simulink model "main_sim_adapt_Gref_SPPH"  (Simulink 7.2)
settings: Solver=ode2  SolverMode=SingleTasking  StartTime=0.0  StopTime=tsim_max  FixedStep=dtsim  RelTol=1e-3
StopFcn:
  | %mkplt
values from neighbouring files (symbols this model uses):
  assertion_time = inf    [setup_taem_sgs_al.m]
  cosA = cos(rwyAZ_rad)    [setup_taem_sgs_al.m]
  E_rwy = E_origin + (mod(( rwyLLA(2)/constants.r2d - lon_origin )+pi,2*pi)-pi) * constants.earth_radius * cos(lat_origin)    [setup_taem_sgs_al.m]
  eow_boundary = tmp_eow(ix(1))    [setup_taem_sgs_al.m]
  N_rwy = N_origin + (mod(( rwyLLA(1)/constants.r2d - lat_origin )+pi,2*pi)-pi) * constants.earth_radius    [setup_taem_sgs_al.m]
  sinA = sin(rwyAZ_rad)    [setup_taem_sgs_al.m]
  vel = 487.2512    [doit.m]
undefined symbols (not defined in the file or in its folder): accel_cmd, aero_surf_qbar_off, aero_surf_qbar_on, Alon, att_cmd_select, att_trim_IC, att_type, att_type_numbers, B1, bb_ellipsoid, bb_params, Blon, C, CA, chi_trim_IC, Clon, command_time, compute_all_rate_cols, compute_all_vel_cols, constants, da_trim_IC, dc_L2W_IC, de_trim_IC, DiscIntNeverNeededParam, dr_trim_IC, dtsim, DZkx, DZtheta, E_trim_IC, Ed_cmd, Ed_trim_IC, fc, flag_uad, full_surf_llim, full_surf_ulim, gain_set, gain_var_struct, gam_cmd_descent, gam_cmd_preflare, gamdot_cmd_descent, gamdot_cmd_flare, gamdot_cmd_preflare, gamma_trim_IC, Gamtheta, Gamx, h_trim_IC, hd_cmd, hd_trim_IC, ideal_vel_Kb, in_exsig_vecin, in_exsig_vecout, invCB, Kb, Kxhat0, Kxnom, Kxstar, lonxm0, MACH, MACH_att_fb, MACH_att_int_IC ... (+77)
libraries: simulink x36, utility_lib x36, mach_lib x24, model_lib x15, simulink_need_slupdate x8, models x6
(part 3 of 7)

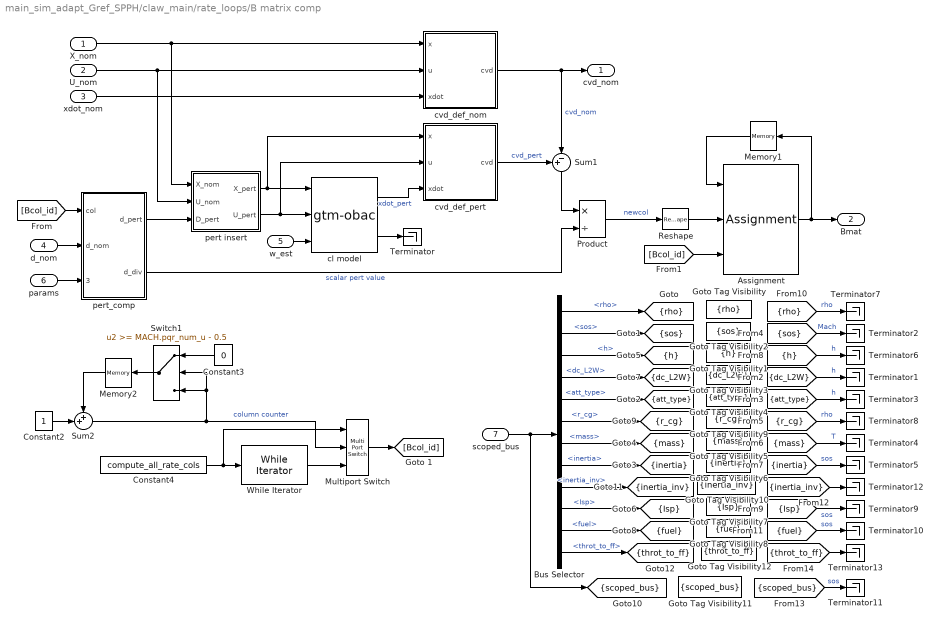
== system main_sim_adapt_Gref_SPPH/claw_main/rate_loops/B matrix comp ==
  X_nom : Inport  OutDataType=sfix(16)  OutScaling=2^0
  U_nom : Inport  Port=2  OutDataType=sfix(16)  OutScaling=2^0
  xdot_nom : Inport  Port=3  OutDataType=sfix(16)  OutScaling=2^0
  d_nom : Inport  Port=4  OutDataType=sfix(16)  OutScaling=2^0
  w_est : Inport  Port=5  OutDataType=sfix(16)  OutScaling=2^0
  params : Inport  Port=6  OutDataType=sfix(16)  OutScaling=2^0
  scoped_bus : Inport  Port=7  OutDataType=sfix(16)  OutScaling=2^0
  Assignment : Assignment  NumberOfDimensions=2  IndexOptions=Assign all,Index vector (port)  Indices=-1,1  OutputSizes=1,1
  Bus Selector : BusSelector  OutputSignals=atmos_env.rho,atmos_env.sos,atmos_env.h,dc_L2W,att_type,mass_props.r_cg,mass_props.mass,mass_props.inertia,mass_props.inertia_inv,mass_props.Isp,mass_props.fuel,mass_props.throt_to_ff
  Constant2 : Constant  OutDataType=sfix(16)  OutScaling=2^0
  Constant3 : Constant  Orientation=left  Value=0  OutDataType=sfix(16)  OutScaling=2^0
  Constant4 : Constant  Value=compute_all_rate_cols  OutDataType=sfix(16)  OutScaling=2^0
  Goto Tag Visibility : GotoTagVisibility  GotoTag=rho
  Goto Tag Visibility1 : GotoTagVisibility  GotoTag=h
  Goto Tag Visibility10 : GotoTagVisibility  GotoTag=inertia_inv
  Goto Tag Visibility11 : GotoTagVisibility  GotoTag=scoped_bus
  Goto Tag Visibility12 : GotoTagVisibility  GotoTag=throt_to_ff
  Goto Tag Visibility2 : GotoTagVisibility  GotoTag=sos
  Goto Tag Visibility3 : GotoTagVisibility  GotoTag=dc_L2W
  Goto Tag Visibility4 : GotoTagVisibility  GotoTag=att_type
  Goto Tag Visibility5 : GotoTagVisibility  GotoTag=mass
  Goto Tag Visibility6 : GotoTagVisibility  GotoTag=inertia
  Goto Tag Visibility7 : GotoTagVisibility  GotoTag=Isp
  Goto Tag Visibility8 : GotoTagVisibility  GotoTag=fuel
  Goto Tag Visibility9 : GotoTagVisibility  GotoTag=r_cg
  Memory1 : Memory  Orientation=left  X0=MACH_pqr_Bmat_IC  InheritSampleTime=on
  Memory2 : Memory  Orientation=left  InheritSampleTime=on
  Multiport Switch : MultiPortSwitch  Inputs=2  zeroidx=on
  Product : Product  Inputs=*/  OutDataType=sfix(16)  OutScaling=2^0  SaturateOnIntegerOverflow=on  InputSameDT=on  OutDataTypeStr=Inherit: Same as first input
  Reshape : Reshape  OutputDimensionality=Column vector (2-D)
  Sum1 : Sum  Orientation=down  Inputs=+-|  OutDataType=sfix(16)  OutScaling=2^0  SaturateOnIntegerOverflow=on  InputSameDT=on  OutDataTypeStr=Inherit: Same as first input
  Sum2 : Sum  Inputs=++|  OutDataType=sfix(16)  OutScaling=2^0  SaturateOnIntegerOverflow=on  InputSameDT=on  OutDataTypeStr=Inherit: Same as first input
  Switch1 : Switch  Orientation=left  Threshold=MACH.pqr_num_u - 0.5  SaturateOnIntegerOverflow=on  InputSameDT=on
  Terminator{,1..13} (14 alike) : Terminator
  While Iterator : WhileIterator  MaxIters=MACH.pqr_num_u  WhileBlockType=do-while  ShowIterationPort=on
  cl model : models/gtm-obac  SystemSampleTime=-1
  cvd_def_nom : Subsystem
  cvd_def_pert : Subsystem
  pert insert : Subsystem
  pert_comp : Subsystem
  cvd_nom : Outport  OutDataType=sfix(16)  OutScaling=2^0
  Bmat : Outport  Port=2  OutDataType=sfix(16)  OutScaling=2^0
  tag scope: Isp=scoped, att_type=scoped, dc_L2W=scoped, fuel=scoped, h=scoped, inertia=scoped, inertia_inv=scoped, mass=scoped, r_cg=scoped, rho=scoped, scoped_bus=scoped, sos=scoped, throt_to_ff=scoped
  wires:
  Reshape/1 -> Assignment/2
  pert_comp/1(d_pert) -> pert insert/3(D_pert)
  pert insert/1(X_pert) -> cvd_def_pert/1(x), cl model/1
  pert insert/2(U_pert) -> cvd_def_pert/2(u), cl model/2
  pert_comp/2(d_div) -> Product/2  "scalar pert value"
  [Bcol_id] -> pert_comp/1(col)
  Assignment/1 -> Bmat/1, Memory1/1
  [Bcol_id] -> Assignment/3
  Sum1/1 -> Product/1
  Product/1 -> Reshape/1  "newcol"
  X_nom/1 -> cvd_def_nom/1(x), pert insert/1(X_nom)
  U_nom/1 -> cvd_def_nom/2(u), pert insert/2(U_nom)
  xdot_nom/1 -> cvd_def_nom/3(xdot)
  cvd_def_pert/1(cvd) -> Sum1/1  "cvd_pert"
  cvd_def_nom/1(cvd) -> Sum1/2, cvd_nom/1  "cvd_nom"
  cl model/1 -> cvd_def_pert/3(xdot)  "xdot_pert"
  w_est/1 -> cl model/3
  d_nom/1 -> pert_comp/2(d_nom)
  Memory1/1 -> Assignment/1
  cl model/2 -> Terminator/1
  params/1 -> pert_comp/3(params)
  Constant4/1 -> Multiport Switch/1, While Iterator/1
  While Iterator/1 -> Multiport Switch/3
  Constant3/1 -> Switch1/1
  Sum2/1 -> Switch1/3, Switch1/2, Multiport Switch/2  "column counter"
  Switch1/1 -> Memory2/1
  Memory2/1 -> Sum2/1
  Constant2/1 -> Sum2/2
  Multiport Switch/1 -> [Bcol_id]
  scoped_bus/1 -> Bus Selector/1, [scoped_bus]
  [rho] -> Terminator7/1  "rho"
  [sos] -> Terminator2/1  "Mach"
  [h] -> Terminator6/1  "h"
  Bus Selector/1 -> [rho]  "<rho>"
  Bus Selector/2 -> [sos]  "<sos>"
  Bus Selector/3 -> [h]  "<h>"
  [dc_L2W] -> Terminator1/1  "h"
  Bus Selector/4 -> [dc_L2W]  "<dc_L2W>"
  [att_type] -> Terminator3/1  "h"
  Bus Selector/5 -> [att_type]  "<att_type>"
  [r_cg] -> Terminator8/1  "rho"
  [mass] -> Terminator4/1  "T"
  [inertia] -> Terminator5/1  "sos"
  Bus Selector/6 -> [r_cg]  "<r_cg>"
  Bus Selector/7 -> [mass]  "<mass>"
  Bus Selector/8 -> [inertia]  "<inertia>"
  [Isp] -> Terminator9/1  "sos"
  Bus Selector/10 -> [Isp]  "<Isp>"
  [fuel] -> Terminator10/1  "sos"
  Bus Selector/11 -> [fuel]  "<fuel>"
  [inertia_inv] -> Terminator12/1
  Bus Selector/9 -> [inertia_inv]  "<inertia_inv>"
  [scoped_bus] -> Terminator11/1  "sos"
  [throt_to_ff] -> Terminator13/1
  Bus Selector/12 -> [throt_to_ff]  "<throt_to_ff>"

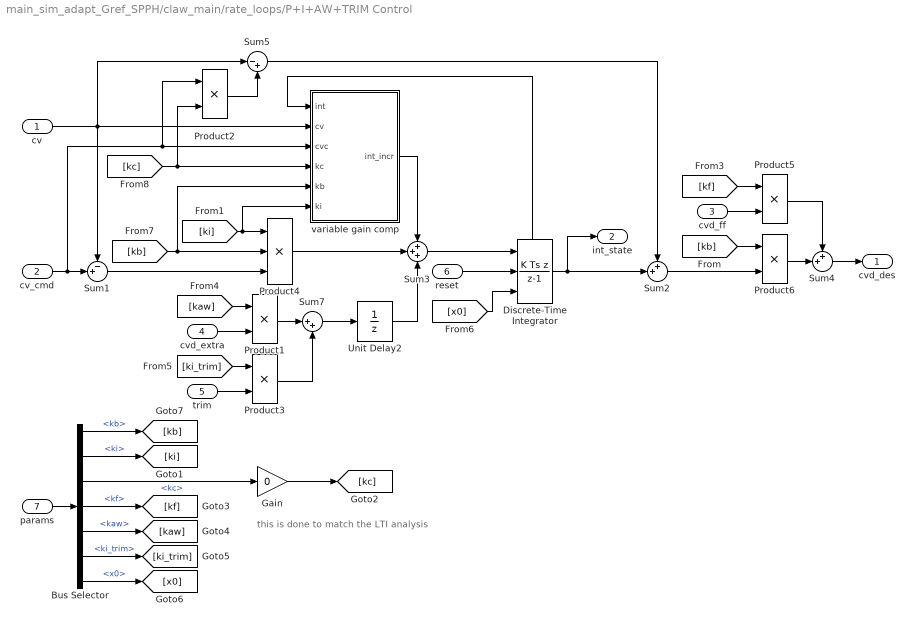
== system main_sim_adapt_Gref_SPPH/claw_main/rate_loops/P+I+AW+TRIM Control ==
  note: this is done to match the LTI analysis
  cv : Inport  OutDataType=sfix(16)  OutScaling=2^0
  cv_cmd : Inport  Port=2  OutDataType=sfix(16)  OutScaling=2^0
  cvd_ff : Inport  Port=3  OutDataType=sfix(16)  OutScaling=2^0
  cvd_extra : Inport  Port=4  OutDataType=sfix(16)  OutScaling=2^0
  trim : Inport  Port=5  OutDataType=sfix(16)  OutScaling=2^0
  reset : Inport  Port=6  OutDataType=sfix(16)  OutScaling=2^0
  params : Inport  Port=7  OutDataType=sfix(16)  OutScaling=2^0
  Bus Selector : BusSelector  OutputSignals=kb,ki,kc,kf,kaw,ki_trim,x0
  Discrete-Time Integrator : DiscreteIntegrator  IntegratorMethod=Integration: Backward Euler  ExternalReset=rising  InitialConditionSource=external  SampleTime=-1  OutDataType=sfix(16)  OutScaling=2^0  ShowStatePort=on  ICPrevOutput=DiscIntNeverNeededParam  ICPrevScaledInput=DiscIntNeverNeededParam
  Gain : Gain  Gain=0  ParameterDataType=sfix(16)  ParameterScaling=2^0  OutDataType=sfix(16)  OutScaling=2^0
  Product{1..3,5..6} (5 alike) : Product  OutDataType=sfix(16)  OutScaling=2^0  RndMeth=Zero
  Product4 : Product  Inputs=3  OutDataType=sfix(16)  OutScaling=2^0  RndMeth=Zero
  Sum1 : Sum  Inputs=-+|  OutDataType=sfix(16)  OutScaling=2^0  SaturateOnIntegerOverflow=on  InputSameDT=on  OutDataTypeStr=Inherit: Same as first input
  Sum2 : Sum  Inputs=++|  OutDataType=sfix(16)  OutScaling=2^0  SaturateOnIntegerOverflow=on  InputSameDT=on  OutDataTypeStr=Inherit: Same as first input
  Sum3 : Sum  Inputs=+++  OutDataType=sfix(16)  OutScaling=2^0  SaturateOnIntegerOverflow=on  InputSameDT=on  OutDataTypeStr=Inherit: Same as first input
  Sum4 : Sum  Inputs=++|  OutDataType=sfix(16)  OutScaling=2^0  SaturateOnIntegerOverflow=on  InputSameDT=on  OutDataTypeStr=Inherit: Same as first input
  Sum5 : Sum  Inputs=|-+  OutDataType=sfix(16)  OutScaling=2^0  SaturateOnIntegerOverflow=on  InputSameDT=on  OutDataTypeStr=Inherit: Same as first input
  Sum7 : Sum  Inputs=|++  OutDataType=sfix(16)  OutScaling=2^0  SaturateOnIntegerOverflow=on  InputSameDT=on  OutDataTypeStr=Inherit: Same as first input
  Unit Delay2 : UnitDelay  SampleTime=-1
  variable gain comp : Subsystem
  cvd_des : Outport  OutDataType=sfix(16)  OutScaling=2^0
  int_state : Outport  Port=2  OutDataType=sfix(16)  OutScaling=2^0
  wires:
  cv_cmd/1 -> Sum1/2, Product2/1, variable gain comp/3(cvc)
  [kb] -> variable gain comp/5(kb), Product4/2
  Sum5/1 -> Sum2/1
  Product2/1 -> Sum5/2
  [kc] -> Product2/2, variable gain comp/4(kc)
  Discrete-Time Integrator/State -> variable gain comp/1(int)
  variable gain comp/1(int_incr) -> Sum3/1
  Product4/1 -> Sum3/2
  Sum2/1 -> Product6/2
  cv/1 -> variable gain comp/2(cv), Sum5/1, Sum1/1
  Bus Selector/7 -> [x0]  "<x0>"
  params/1 -> Bus Selector/1
  [kf] -> Product5/1
  cvd_ff/1 -> Product5/2
  [kb] -> Product6/1
  [ki] -> variable gain comp/6(ki), Product4/1
  Sum1/1 -> Product4/3
  [ki_trim] -> Product3/1
  Product1/1 -> Sum7/1
  [kaw] -> Product1/1
  Bus Selector/6 -> [ki_trim]  "<ki_trim>"
  Bus Selector/5 -> [kaw]  "<kaw>"
  Bus Selector/4 -> [kf]  "<kf>"
  Bus Selector/3 -> Gain/1  "<kc>"
  Bus Selector/2 -> [ki]  "<ki>"
  Bus Selector/1 -> [kb]  "<kb>"
  Sum7/1 -> Unit Delay2/1
  Product3/1 -> Sum7/2
  reset/1 -> Discrete-Time Integrator/2
  cvd_extra/1 -> Product1/2
  Discrete-Time Integrator/1 -> Sum2/2, int_state/1
  Sum3/1 -> Discrete-Time Integrator/1
  Unit Delay2/1 -> Sum3/3
  trim/1 -> Product3/2
  Product6/1 -> Sum4/2
  Sum4/1 -> cvd_des/1
  Product5/1 -> Sum4/1
  [x0] -> Discrete-Time Integrator/3
  Gain/1 -> [kc]

== system main_sim_adapt_Gref_SPPH/claw_main/rate_loops/allocation ==
  cvd_nom : Inport  OutDataType=sfix(16)  OutScaling=2^0
  Bmat : Inport  Port=2  OutDataType=sfix(16)  OutScaling=2^0
  d_old : Inport  Port=3  OutDataType=sfix(16)  OutScaling=2^0
  d_nom : Inport  Port=4  OutDataType=sfix(16)  OutScaling=2^0
  cvd_des : Inport  Port=5  OutDataType=sfix(16)  OutScaling=2^0
  params : Inport  Port=6  OutDataType=sfix(16)  OutScaling=2^0
  Bmat_rcs : Selector  NumberOfDimensions=2  InputPortWidth=MACH.num_u  IndexOptions=Select all,Index vector (dialog)  Indices=-1,MACH.pqr_u_rcs_idx  OutputSizes=1
  Bmat_smn : Selector  NumberOfDimensions=2  InputPortWidth=MACH.num_u  IndexOptions=Select all,Index vector (dialog)  Indices=-1,MACH.pqr_u_smn_idx  OutputSizes=1
  Gain : Gain  Gain=-1  ParameterDataType=sfix(16)  ParameterScaling=2^0  OutDataType=sfix(16)  OutScaling=2^0
  Mux3 : Mux  Inputs=2
  RCS allocation : Subsystem
  Selector : Selector  NumberOfDimensions=2  InputPortWidth=MACH.num_u  IndexOptions=Index vector (dialog),Index vector (dialog)  Indices=1:9,1:2  OutputSizes=1
  config_di : Subsystem  BlockChoice=di_smn  mask{num_cv=MACH.pqr_num_cv, num_u=MACH.pqr_num_u_smn, wght_cv_type=MACH.pqr_wght_cv_type}
      link override di_smn/config_smn/smn_sfunc: sfunc_name=MACH.smn_sfunc_name
      settings: AttributesFormatString=%<BlockChoice>  TemplateBlock=mach_lib/config_di  MemberBlocks=di_pseudoinv,di_smn
  d_nom_smn : Selector  InputPortWidth=MACH.pqr_num_u  IndexOptions=Index vector (dialog)  Indices=MACH.pqr_u_smn_idx  OutputSizes=1
  d_old_rcs : Selector  InputPortWidth=MACH.pqr_num_u  IndexOptions=Index vector (dialog)  Indices=MACH.pqr_u_rcs_idx  OutputSizes=1
  d_old_smn : Selector  InputPortWidth=MACH.pqr_num_u  IndexOptions=Index vector (dialog)  Indices=MACH.pqr_u_smn_idx  OutputSizes=1
  param select rcs : Subsystem  mask{idx=MACH.pqr_u_rcs_idx}
      mask prompts: idx "index"
  param select smn : Subsystem  mask{idx=MACH.pqr_u_smn_idx}
      mask prompts: idx "index"
  d_cmd : Outport  OutDataType=sfix(16)  OutScaling=2^0
  cvd_extra_smn : Outport  Port=2  OutDataType=sfix(16)  OutScaling=2^0
  lambda : Outport  Port=3  OutDataType=sfix(16)  OutScaling=2^0
  solve_dat : Outport  Port=4  OutDataType=sfix(16)  OutScaling=2^0
  cvd_extra : Outport  Port=5  OutDataType=sfix(16)  OutScaling=2^0
  wires:
  config_di/1(d_cmd) -> Mux3/1
  d_nom_smn/1 -> config_di/4(d_nom)
  d_old_smn/1 -> config_di/3(d_old)
  Bmat_rcs/1 -> RCS allocation/1(Bmat)
  [Bmat] -> Bmat_rcs/1
  RCS allocation/1(rcs_cmd) -> Mux3/2
  d_old_rcs/1 -> RCS allocation/2(rcs_cmd_old)
  Bmat_smn/1 -> config_di/2(Bmat)
  Gain/1 -> RCS allocation/3(cvd_des)
  [d_old] -> d_old_rcs/1
  config_di/2(cvd_extra) -> Gain/1, cvd_extra_smn/1  "cvdex_smn"
  config_di/4(solve_dat) -> Selector/1
  cvd_nom/1 -> config_di/1(cvd_nom)
  Bmat/1 -> Bmat_smn/1, [Bmat]
  d_nom/1 -> d_nom_smn/1
  Mux3/1 -> d_cmd/1
  d_old/1 -> d_old_smn/1, [d_old]
  config_di/3(lambda) -> lambda/1
  cvd_des/1 -> config_di/5(cvd_des)
  RCS allocation/2(cvd_extra) -> cvd_extra/1
  param select smn/1(params) -> config_di/6(params)
  Selector/1 -> solve_dat/1
  params/1 -> param select smn/1(params_all), param select rcs/1(params_all)
  param select rcs/1(params) -> RCS allocation/4(params)

== system main_sim_adapt_Gref_SPPH/claw_main/rate_loops/bangbang ==
  enable_bb : Inport  OutDataType=sfix(16)  OutScaling=2^0
  att_cvc : Inport  Port=2  OutDataType=sfix(16)  OutScaling=2^0
  att_cv : Inport  Port=3  OutDataType=sfix(16)  OutScaling=2^0
  pqr : Inport  Port=4  OutDataType=sfix(16)  OutScaling=2^0
  cvd_des_lin : Inport  Port=5  OutDataType=sfix(16)  OutScaling=2^0
  Bang Bang : Stateflow chart
  Constant1 : Constant  Value=bb_params  OutDataType=sfix(16)  OutScaling=2^0
  Constant2 : Constant  Value=bb_ellipsoid  OutDataType=sfix(16)  OutScaling=2^0
  Mux : Mux  Inputs=[12 3 3 1 1 3]
  Unit Delay : UnitDelay  X0=[ 0 0 0 ]  SampleTime=MACH.dt
  Unit Delay1 : UnitDelay  SampleTime=MACH.dt
  Unit Delay2 : UnitDelay  SampleTime=MACH.dt
  cvd_des : Outport  OutDataType=sfix(16)  OutScaling=2^0
  bb_debug : Outport  Port=2  OutDataType=sfix(16)  OutScaling=2^0
  wires:
  att_cvc/1 -> Bang Bang/3(att_cvc)
  pqr/1 -> Bang Bang/5(pqr)
  att_cv/1 -> Bang Bang/4(att_cv)
  Unit Delay1/1 -> Bang Bang/11(timer_old)
  Bang Bang/5(timer) -> Unit Delay1/1, Mux/5
  Bang Bang/3(dir) -> Unit Delay/1, Mux/3
  Unit Delay/1 -> Bang Bang/9(dir_old)
  Constant1/1 -> Bang Bang/1(bb_params)
  [inertia] -> Bang Bang/6(inertia)
  enable_bb/1 -> Bang Bang/7(enable_bb)
  Unit Delay2/1 -> Bang Bang/10(use_bb_old)
  Bang Bang/4(use_bb) -> Unit Delay2/1, Mux/4
  cvd_des_lin/1 -> Bang Bang/8(cvddes_lin), Mux/6  "cvd_des_lin"
  Constant2/1 -> Bang Bang/2(bb_ellipsoid)
  Bang Bang/1(debug_output) -> Mux/1
  Mux/1 -> bb_debug/1
  Bang Bang/2(cvddes) -> cvd_des/1, Mux/2  "cvd_des"

== system main_sim_adapt_Gref_SPPH/claw_main/rate_loops/compute trim ==
  inner cmd : Inport  OutDataType=sfix(16)  OutScaling=2^0
  Bmat : Inport  Port=2  OutDataType=sfix(16)  OutScaling=2^0
  cmd : Inport  Port=3  OutDataType=sfix(16)  OutScaling=2^0
  Product : Product  Multiplication=Matrix(*)  OutDataType=sfix(16)  OutScaling=2^0  SaturateOnIntegerOverflow=on  OutDataTypeStr=Inherit: Same as first input
  Sum1 : Sum  Inputs=|+-  OutDataType=sfix(16)  OutScaling=2^0  SaturateOnIntegerOverflow=on
  trim : Outport  OutDataType=sfix(16)  OutScaling=2^0
  wires:
  Product/1 -> trim/1
  Bmat/1 -> Product/1
  Sum1/1 -> Product/2
  inner cmd/1 -> Sum1/1
  cmd/1 -> Sum1/2

== system main_sim_adapt_Gref_SPPH/claw_main/rate_loops/select rate cmd ==
  pqr_current : Inport  OutDataType=sfix(16)  OutScaling=2^0
  throt_current : Inport  Port=2  OutDataType=sfix(16)  OutScaling=2^0
  outer cmd : Inport  Port=3  OutDataType=sfix(16)  OutScaling=2^0
  signal_bus : Inport  Port=4  OutDataType=sfix(16)  OutScaling=2^0
  Bus Selector6 : BusSelector  OutputSignals=cmd_bus.select_cmd.rate
  Demux : Demux  Outputs=[ MACH.pqr_num_cv MACH.num_u_throt ]
  Multiport Switch : MultiPortSwitch  zeroidx=on  SaturateOnIntegerOverflow=on
  Mux1 : Mux  Inputs=2
  Unit Delay1 : UnitDelay  X0=MACH_throttle_IC  SampleTime=-1
  get direct cmd : Subsystem
  select multiple throts : Selector  InputPortWidth=4  IndexOptions=Index vector (dialog)  Indices=[1:3 4*ones(1,MACH.num_u_throt)]  OutputSizes=1
  pqr_cmd : Outport  OutDataType=sfix(16)  OutScaling=2^0
  throt_cmd : Outport  Port=2  OutDataType=sfix(16)  OutScaling=2^0
  cmd : Outport  Port=3  OutDataType=sfix(16)  OutScaling=2^0
  wires:
  Multiport Switch/1 -> cmd/1, Demux/1
  outer cmd/1 -> Multiport Switch/4
  Mux1/1 -> Multiport Switch/2
  select multiple throts/1 -> Multiport Switch/1
  Unit Delay1/1 -> Mux1/2
  pqr_current/1 -> Mux1/1
  throt_current/1 -> Unit Delay1/1
  get direct cmd/1(direct_cmd) -> Multiport Switch/3
  signal_bus/1 -> get direct cmd/1(signal_bus), Bus Selector6/1
  Bus Selector6/1 -> select multiple throts/1  "<rate>"
  Demux/1 -> pqr_cmd/1
  Demux/2 -> throt_cmd/1

== system main_sim_adapt_Gref_SPPH/claw_main/rate_loops/set rate loop params ==
  rate_params : Inport  OutDataType=sfix(16)  OutScaling=2^0
  u_old : Inport  Port=2  OutDataType=sfix(16)  OutScaling=2^0
  Bus Assignment : BusAssignment  AssignedSignals=u_ulim,u_llim
  Bus Selector1 : BusSelector  OutputSignals=u_ulim,u_llim,u_urlim,u_lrlim
  rate limit limits : mach_lib/rate limit limits  SystemSampleTime=-1  ulim=MACH.pqr_u_ulim  llim=MACH.pqr_u_llim
  params : Outport  OutDataType=sfix(16)  OutScaling=2^0
  wires:
  u_old/1 -> rate limit limits/1
  rate_params/1 -> Bus Selector1/1, Bus Assignment/1
  Bus Selector1/1 -> rate limit limits/2  "<u_ulim>"
  Bus Selector1/2 -> rate limit limits/3  "<u_llim>"
  Bus Selector1/3 -> rate limit limits/4  "<u_urlim>"
  Bus Selector1/4 -> rate limit limits/5  "<u_lrlim>"
  rate limit limits/1 -> Bus Assignment/2
  rate limit limits/2 -> Bus Assignment/3
  Bus Assignment/1 -> params/1

== system main_sim_adapt_Gref_SPPH/claw_main/servo commands  when not engaged/pseudo surf cmd ==
  autopilot_cmd : Inport  OutDataType=sfix(16)  OutScaling=2^0
  Assignment1 : Assignment  IndexOptions=Index vector (dialog)  Indices=[ MACH.vane_idx MACH.throttle_idx ]  OutputSizes=[1 1]
  Constant : Constant  Value=MACH_U_nom_IC  OutDataType=sfix(16)  OutScaling=2^0
  Demux2 : Demux  Outputs=[ 3 1 ]
  Gain : Gain  Gain=MACH.mixer  Multiplication=Matrix(K*u)  ParameterDataType=sfix(16)  ParameterScaling=2^0  OutDataType=sfix(16)  OutScaling=2^0  SaturateOnIntegerOverflow=on  OutDataTypeStr=Inherit: Same as input  ParamDataTypeStr=Inherit: Same as input
  Gain1 : Gain  Gain=MACH.throt_mixer  ParameterDataType=sfix(16)  ParameterScaling=2^0  OutDataType=sfix(16)  OutScaling=2^0
  Mux : Mux  Inputs=2
  surf_cmd : Outport  OutDataType=sfix(16)  OutScaling=2^0
  wires:
  Mux/1 -> Assignment1/2
  Gain1/1 -> Mux/2
  Gain/1 -> Mux/1
  Demux2/2 -> Gain1/1  "throttle"
  Demux2/1 -> Gain/1  "da,de,dr"
  autopilot_cmd/1 -> Demux2/1
  Assignment1/1 -> surf_cmd/1
  Constant/1 -> Assignment1/1

== system main_sim_adapt_Gref_SPPH/claw_main/state est/process inputs ==
  u_old : Inport  OutDataType=sfix(16)  OutScaling=2^0
  sensors : Inport  Port=2  OutDataType=sfix(16)  OutScaling=2^0
  Bus Selector2 : BusSelector  OutputSignals=u_meas
  Constant : Constant  Value=0  OutDataType=sfix(16)  OutScaling=2^0
  Multiport Switch1 : MultiPortSwitch  Inputs=2  zeroidx=on  SaturateOnIntegerOverflow=on
  throt : Selector  InputPortWidth=MACH.num_u  IndexOptions=Index vector (dialog)  Indices=MACH.throttle_idx  OutputSizes=1
  use throt estimate from measurement instead of past throt cmd : Assignment  IndexOptions=Index vector (dialog)  Indices=MACH.throttle_idx  OutputSizes=[1 1]
  use_throt_estimate : Constant  Value=use_throt_estimate  OutDataType=sfix(16)  OutScaling=2^0
  zero RCS inputs : Assignment  IndexOptions=Index vector (dialog)  Indices=MACH.rcs_idx  OutputSizes=[1 1]
  u_est : Outport  OutDataType=sfix(16)  OutScaling=2^0
  wires:
  u_old/1 -> use throt estimate from measurement instead of past throt cmd/1, Multiport Switch1/2
  use_throt_estimate/1 -> Multiport Switch1/1
  use throt estimate from measurement instead of past throt cmd/1 -> Multiport Switch1/3
  sensors/1 -> Bus Selector2/1
  Bus Selector2/1 -> throt/1  "<u_meas>"
  Multiport Switch1/1 -> zero RCS inputs/1
  Constant/1 -> zero RCS inputs/2
  zero RCS inputs/1 -> u_est/1
  throt/1 -> use throt estimate from measurement instead of past throt cmd/2

== system main_sim_adapt_Gref_SPPH/claw_main/state est/process sensors ==
  reset_pos : Inport  OutDataType=sfix(16)  OutScaling=2^0
  nav_ok : Inport  Port=2  OutDataType=sfix(16)  OutScaling=2^0
  pqr : Inport  Port=3  OutDataType=sfix(16)  OutScaling=2^0
  NED_dot : Inport  Port=4  OutDataType=sfix(16)  OutScaling=2^0
  latlonh : Inport  Port=5  OutDataType=sfix(16)  OutScaling=2^0
  e : Inport  Port=6  OutDataType=sfix(16)  OutScaling=2^0
  Bus Creator : BusCreator
  Gain : Gain  Gain=[1 1 -1]  ParameterDataType=sfix(16)  ParameterScaling=2^0  OutDataType=sfix(16)  OutScaling=2^0  SaturateOnIntegerOverflow=on  OutDataTypeStr=Inherit: Same as input  ParamDataTypeStr=Inherit: Same as input
  Gain1 : Gain  Gain=[1 1 0]  ParameterDataType=sfix(16)  ParameterScaling=2^0  OutDataType=sfix(16)  OutScaling=2^0  SaturateOnIntegerOverflow=on  OutDataTypeStr=Inherit: Same as input  ParamDataTypeStr=Inherit: Same as input
  LLh2NEh : utility_lib/LLh2NEh  SystemSampleTime=-1
  Product : Product  Multiplication=Matrix(*)  OutDataType=sfix(16)  OutScaling=2^0  SaturateOnIntegerOverflow=on  OutDataTypeStr=Inherit: Same as first input
  Reshape : Reshape  OutputDimensionality=Customize  OutputDimensions=[3,3]
  Selector : Selector  InputPortWidth=3  IndexOptions=Index vector (dialog)  Indices=[3]  OutputSizes=1
  Sum : Sum  Inputs=|+-  OutDataType=sfix(16)  OutScaling=2^0  SaturateOnIntegerOverflow=on
  Switch1 : Switch  Threshold=0.5  SaturateOnIntegerOverflow=on
  Switch2 : Switch  Threshold=0.5  SaturateOnIntegerOverflow=on
  Unit Delay : UnitDelay  Orientation=left  SampleTime=-1
  Unit Delay1 : UnitDelay  Orientation=left  X0=MACH_quat_IC  SampleTime=-1
  compute dc_fltpath : Subsystem
  e2dc : utility_lib/e2dc  SystemSampleTime=-1
  navigation complementary filter : Subsystem
  select e sign : Subsystem
  use_nav : Constant  Value=use_nav  OutDataType=sfix(16)  OutScaling=2^0
  wait for valid nav : Subsystem
  vehicle_origin : Outport  OutDataType=sfix(16)  OutScaling=2^0
  h_geodetic : Outport  Port=2  OutDataType=sfix(16)  OutScaling=2^0
  NEh_nav : Outport  Port=3  OutDataType=sfix(16)  OutScaling=2^0
  nav_valid : Outport  Port=4  OutDataType=sfix(16)  OutScaling=2^0
  NEh_dot : Outport  Port=5  OutDataType=sfix(16)  OutScaling=2^0
  dc_fltpath : Outport  Port=6  OutDataType=sfix(16)  OutScaling=2^0
  cvc_origin : Outport  Port=7  OutDataType=sfix(16)  OutScaling=2^0
  dircos : Outport  Port=8  OutDataType=sfix(16)  OutScaling=2^0
  x_est : Outport  Port=9  OutDataType=sfix(16)  OutScaling=2^0
  wires:
  e/1 -> select e sign/1(e in)
  Unit Delay1/1 -> select e sign/2(e_past)
  wait for valid nav/1(LLh_0) -> Gain1/1
  Sum/1 -> Bus Creator/3  "NEh"
  navigation complementary filter/1(NEh_fil) -> Switch2/3
  use_nav/1 -> Switch2/2
  Switch2/1 -> Sum/1, NEh_nav/1, Switch1/1
  Unit Delay/1 -> Switch1/3
  Switch1/1 -> Unit Delay/1, cvc_origin/1, Sum/2  "NEh"
  LLh2NEh/1 -> navigation complementary filter/1(NEh nav), Switch2/1
  wait for valid nav/2(nav_valid) -> nav_valid/1
  nav_ok/1 -> wait for valid nav/2(nav_ok)
  reset_pos/1 -> Switch1/2
  latlonh/1 -> wait for valid nav/1(latlonh), LLh2NEh/1, Selector/1
  e2dc/1 -> dircos/1, Reshape/1
  NED_dot/1 -> Product/2, Gain/1
  Gain/1 -> navigation complementary filter/2(NEh dot), compute dc_fltpath/1(NEh_dot_fltpath), NEh_dot/1
  select e sign/1(e out) -> Unit Delay1/1, e2dc/1, Bus Creator/4  "e"
  Reshape/1 -> Product/1
  pqr/1 -> Bus Creator/1  "pqr"
  Product/1 -> Bus Creator/2  "uvw"
  Bus Creator/1 -> x_est/1
  Selector/1 -> h_geodetic/1
  Gain1/1 -> LLh2NEh/2, vehicle_origin/1
  compute dc_fltpath/1(dc_fltpath) -> dc_fltpath/1

== system main_sim_adapt_Gref_SPPH/claw_main/state est/wind estimator ==
  dircos : Inport  OutDataType=sfix(16)  OutScaling=2^0
  x : Inport  Port=2  OutDataType=sfix(16)  OutScaling=2^0
  sensors : Inport  Port=3  OutDataType=sfix(16)  OutScaling=2^0
  u : Inport  Port=4  OutDataType=sfix(16)  OutScaling=2^0
  wind_est_sw : Inport  Port=5  OutDataType=sfix(16)  OutScaling=2^0
  Bus Selector1 : BusSelector  OutputSignals=NED_wind,accels_cg
  Bus Selector2 : BusSelector  OutputSignals=accels_cg
  Multiport Switch1 : MultiPortSwitch  Inputs=2  zeroidx=on  SaturateOnIntegerOverflow=on
  Unit Delay : UnitDelay  X0=zeros(3,1)  SampleTime=-1
  cl model : models/gtm-obac  SystemSampleTime=-1
  use_wind_est : Constant  Value=use_wind_est  OutDataType=sfix(16)  OutScaling=2^0
  wind estimate : Subsystem
  w_est : Outport  OutDataType=sfix(16)  OutScaling=2^0
  w_est_debug : Outport  Port=2  OutDataType=sfix(16)  OutScaling=2^0
  wires:
  cl model/1 -> wind estimate/3(xdot)
  Unit Delay/1 -> cl model/3
  use_wind_est/1 -> Multiport Switch1/1
  wind estimate/1(w_est) -> Unit Delay/1, Multiport Switch1/3
  x/1 -> wind estimate/2(x), cl model/1
  u/1 -> cl model/2
  dircos/1 -> wind estimate/1(dircos)
  Multiport Switch1/1 -> w_est/1
  wind_est_sw/1 -> wind estimate/6(wind_est_sw)
  sensors/1 -> Bus Selector1/1
  wind estimate/2(w_est_debug) -> w_est_debug/1
  Bus Selector1/1 -> Multiport Switch1/2  "<NED_wind>"
  Bus Selector1/2 -> wind estimate/5(sensed_accels_cg)  "<accels_cg>"
  cl model/2 -> Bus Selector2/1
  Bus Selector2/1 -> wind estimate/4(model_accels_cg)  "<accels_cg>"

== system main_sim_adapt_Gref_SPPH/claw_main/vel_loops/B matrix comp ==
  note: Note: Ideally,  X_nom and U_nom
      |  would be constructed to be near
      |  moment equalibrium
  X : Inport  OutDataType=sfix(16)  OutScaling=2^0
  U_limited : Inport  Port=2  OutDataType=sfix(16)  OutScaling=2^0
  d_nom : Inport  Port=3  OutDataType=sfix(16)  OutScaling=2^0
  camcmd : Inport  Port=4  OutDataType=sfix(16)  OutScaling=2^0
  params : Inport  Port=5  OutDataType=sfix(16)  OutScaling=2^0
  w_est : Inport  Port=6  OutDataType=sfix(16)  OutScaling=2^0
  NEh_dot : Inport  Port=7  OutDataType=sfix(16)  OutScaling=2^0
  scoped_bus : Inport  Port=8  OutDataType=sfix(16)  OutScaling=2^0
  B matrix comp : Subsystem  TreatAsAtomicUnit=on
  Constant : Constant  Value=0  OutDataType=sfix(16)  OutScaling=2^0
  Constant1 : Constant  Value=0  OutDataType=sfix(16)  OutScaling=2^0
  compute cvd_nom : Subsystem
  compute nominal XU : Subsystem
  zero pqr : Assignment  IndexOptions=Index vector (dialog)  Indices=MACH.pqr_idx  OutputSizes=[1 1]
  zero rate surfs : Assignment  IndexOptions=Index vector (dialog)  Indices=MACH.pqr_u_idx  OutputSizes=[1 1]
  cvd_nom : Outport  OutDataType=sfix(16)  OutScaling=2^0
  Bmat : Outport  Port=2  OutDataType=sfix(16)  OutScaling=2^0
  wires:
  camcmd/1 -> B matrix comp/6(camcmd), compute nominal XU/4(camcmd)
  scoped_bus/1 -> B matrix comp/9(scoped_bus)
  d_nom/1 -> B matrix comp/5(d_nom), compute nominal XU/3(D_in)
  params/1 -> B matrix comp/8(params)
  NEh_dot/1 -> B matrix comp/7(NEh_dot), compute nominal XU/5(NEh_dot)
  compute cvd_nom/1(cvd) -> cvd_nom/1, B matrix comp/1(cvd_nom)
  w_est/1 -> B matrix comp/4(w_est), compute cvd_nom/3(w_est)
  B matrix comp/1(Bmat) -> Bmat/1
  compute nominal XU/1(X_out) -> compute cvd_nom/1(x), B matrix comp/2(X_nom)
  compute nominal XU/2(U_out) -> compute cvd_nom/2(u), B matrix comp/3(U_nom)
  zero rate surfs/1 -> compute nominal XU/2(U_in)
  zero pqr/1 -> compute nominal XU/1(X_in)
  Constant/1 -> zero pqr/2
  Constant1/1 -> zero rate surfs/2
  U_limited/1 -> zero rate surfs/1
  X/1 -> zero pqr/1

== system main_sim_adapt_Gref_SPPH/claw_main/vel_loops/compute trim ==
  inner cmd : Inport  OutDataType=sfix(16)  OutScaling=2^0
  Bmat : Inport  Port=2  OutDataType=sfix(16)  OutScaling=2^0
  cmd : Inport  Port=3  OutDataType=sfix(16)  OutScaling=2^0
  Product : Product  Multiplication=Matrix(*)  OutDataType=sfix(16)  OutScaling=2^0  SaturateOnIntegerOverflow=on  OutDataTypeStr=Inherit: Same as first input
  Sum1 : Sum  Inputs=|+-  OutDataType=sfix(16)  OutScaling=2^0  SaturateOnIntegerOverflow=on
  trim : Outport  OutDataType=sfix(16)  OutScaling=2^0
  wires:
  Product/1 -> trim/1
  Bmat/1 -> Product/1
  Sum1/1 -> Product/2
  inner cmd/1 -> Sum1/1
  cmd/1 -> Sum1/2

== system main_sim_adapt_Gref_SPPH/claw_main/vel_loops/config_di ==
  cvd_nom : Inport  OutDataType=sfix(16)  OutScaling=2^0
  Bmat : Inport  Port=2  OutDataType=sfix(16)  OutScaling=2^0
  d_old : Inport  Port=3  OutDataType=sfix(16)  OutScaling=2^0
  d_nom : Inport  Port=4  OutDataType=sfix(16)  OutScaling=2^0
  cvd_des : Inport  Port=5  OutDataType=sfix(16)  OutScaling=2^0
  params : Inport  Port=6  OutDataType=sfix(16)  OutScaling=2^0
  di_smn : mach_lib/di_smn  SystemSampleTime=-1
  d_cmd : Outport  OutDataType=sfix(16)  OutScaling=2^0
  cvd_extra : Outport  Port=2  OutDataType=sfix(16)  OutScaling=2^0
  lambda : Outport  Port=3  OutDataType=sfix(16)  OutScaling=2^0
  solve_dat : Outport  Port=4  OutDataType=sfix(16)  OutScaling=2^0
  wires:
  cvd_nom/1 -> di_smn/1
  Bmat/1 -> di_smn/2
  d_old/1 -> di_smn/3
  d_nom/1 -> di_smn/4
  cvd_des/1 -> di_smn/5
  params/1 -> di_smn/6
  di_smn/1 -> d_cmd/1
  di_smn/2 -> cvd_extra/1
  di_smn/3 -> lambda/1
  di_smn/4 -> solve_dat/1

== system main_sim_adapt_Gref_SPPH/claw_main/vel_loops/convert accel_cmd to NED_dd_cmd ==
  accel_cmd : Inport  OutDataType=sfix(16)  OutScaling=2^0
  accel_cmd_sw : Inport  Port=2  OutDataType=sfix(16)  OutScaling=2^0
  NEh_d : Inport  Port=3  OutDataType=sfix(16)  OutScaling=2^0
  Merge : Merge  InitialOutput=zeros(3,1)
  MinMax : MinMax  Function=max  OutDataType=sfix(16)  OutScaling=2^0
  NED_dd cmd : Subsystem  TreatAsAtomicUnit=on
  Switch Case : SwitchCase  CaseConditions={1,2}  CaseShowDefault=off
  vchigam_dot cmd : Subsystem  TreatAsAtomicUnit=on
  NEh_dd_cmd : Outport  OutDataType=sfix(16)  OutScaling=2^0
  wires:
  accel_cmd_sw/1 -> MinMax/1
  MinMax/1 -> Switch Case/1
  NEh_d/1 -> vchigam_dot cmd/2(NEh_d)
  vchigam_dot cmd/1(NEh_dd_cmd) -> Merge/2
  Merge/1 -> NEh_dd_cmd/1
  Switch Case/1 -> NED_dd cmd/Action
  Switch Case/2 -> vchigam_dot cmd/Action
  accel_cmd/1 -> vchigam_dot cmd/1(vchigam_dot_cmd), NED_dd cmd/1(NEH_dd_cmd_in)
  NED_dd cmd/1(NEh_dd_cmd) -> Merge/1

== system main_sim_adapt_Gref_SPPH/claw_main/vel_loops/from inner ==
  att,T : Inport  OutDataType=sfix(16)  OutScaling=2^0
  Demux1 : Demux  Outputs=[ 2 1 MACH.num_u_throt ]
  Mux1 : Mux  Inputs=2
  Terminator : Terminator
  d_cmd : Outport  OutDataType=sfix(16)  OutScaling=2^0
  wires:
  att,T/1 -> Demux1/1
  Demux1/1 -> Mux1/1
  Mux1/1 -> d_cmd/1
  Demux1/3 -> Mux1/2
  Demux1/2 -> Terminator/1

== system main_sim_adapt_Gref_SPPH/claw_main/vel_loops/from quat ==
  e,T : Inport  OutDataType=sfix(16)  OutScaling=2^0
  Demux1 : Demux  Outputs=[ 4 MACH.num_u_throt ]
  Mux1 : Mux  Inputs=2
  Selector1 : Selector  InputPortWidth=3  IndexOptions=Index vector (dialog)  Indices=1:2  OutputSizes=1
  e2att : utility_lib/e2att  SystemSampleTime=-1
  d_cmd : Outport  OutDataType=sfix(16)  OutScaling=2^0
  wires:
  e2att/1 -> Selector1/1
  Selector1/1 -> Mux1/1
  Demux1/2 -> Mux1/2
  Mux1/1 -> d_cmd/1
  Demux1/1 -> e2att/1
  e,T/1 -> Demux1/1

== system main_sim_adapt_Gref_SPPH/claw_main/vel_loops/select vel cmd ==
  NEh_dot_current : Inport  OutDataType=sfix(16)  OutScaling=2^0
  cam_current : Inport  Port=2  OutDataType=sfix(16)  OutScaling=2^0
  outer cmd : Inport  Port=3  OutDataType=sfix(16)  OutScaling=2^0
  signal_bus : Inport  Port=4  OutDataType=sfix(16)  OutScaling=2^0
  Bus Selector : BusSelector  OutputSignals=cmd_bus.select_cmd.vel,cmd_bus.autopilot_cmd
  Demux3 : Demux  Outputs=[ MACH.vel_num_cv 1 ]
  Multiport Switch : MultiPortSwitch  zeroidx=on  SaturateOnIntegerOverflow=on
  Mux : Mux  Inputs=2
  Selector1 : Selector  InputPortWidth=4  IndexOptions=Index vector (dialog)  Indices=[1 2 4 3]  OutputSizes=1
  Selector2 : Selector  InputPortWidth=4  IndexOptions=Index vector (dialog)  Indices=[1 2 4 3]  OutputSizes=1
  NEh_dot_cmd : Outport  OutDataType=sfix(16)  OutScaling=2^0
  cam_cmd : Outport  Port=2  OutDataType=sfix(16)  OutScaling=2^0
  cmd : Outport  Port=3  OutDataType=sfix(16)  OutScaling=2^0
  wires:
  Multiport Switch/1 -> cmd/1, Selector2/1
  outer cmd/1 -> Multiport Switch/4
  Bus Selector/1 -> Multiport Switch/1  "<vel>"
  Selector2/1 -> Demux3/1
  Demux3/1 -> NEh_dot_cmd/1
  Demux3/2 -> cam_cmd/1
  Mux/1 -> Selector1/1
  NEh_dot_current/1 -> Mux/1
  Selector1/1 -> Multiport Switch/2
  signal_bus/1 -> Bus Selector/1
  Bus Selector/2 -> Multiport Switch/3  "<autopilot_cmd>"
  cam_current/1 -> Mux/2

== system main_sim_adapt_Gref_SPPH/claw_main/vel_loops/set di params ==
  note: Note: dc_fltpath is now computed from NEh_dot.
      | Switch to recover old computation base on NEh_dot_cmd
  NEh_dot_cmd : Inport  OutDataType=sfix(16)  OutScaling=2^0
  full_surf : Inport  Port=2  OutDataType=sfix(16)  OutScaling=2^0
  u_old : Inport  Port=3  OutDataType=sfix(16)  OutScaling=2^0
  uvw : Inport  Port=4  OutDataType=sfix(16)  OutScaling=2^0
  dc_fltpath : Inport  Port=5  OutDataType=sfix(16)  OutScaling=2^0
  Bus Creator1 : BusCreator  Inputs=7
  Bus Selector : BusSelector  OutputSignals=u_ulim,u_llim,u_urlim,u_lrlim
  Bus Selector1 : BusSelector  OutputSignals=throt_ulim,throt_llim
  Constant1 : Constant  Value=MACH.vel_wght_cv  OutDataType=sfix(16)  OutScaling=2^0
  Constant3 : Constant  Value=MACH.vel_u_pref  OutDataType=sfix(16)  OutScaling=2^0
  Constant4 : Constant  Value=MACH.vel_wght_u_pref  OutDataType=sfix(16)  OutScaling=2^0
  Demux1 : Demux  Outputs=[ 2 MACH.num_u_throt ]
  Gain2 : Gain  Gain=repmat(MACH.vel_wght_fltpath',1,3)  ParameterDataType=sfix(16)  ParameterScaling=2^0  OutDataType=sfix(16)  OutScaling=2^0
  Logical Operator : Logic  Inputs=1  AllPortsSameDT=off  OutDataTypeMode=boolean  OutDataTypeStr=boolean
  Manual Switch : simulink/Signal Routing/Manual Switch  SystemSampleTime=-1  sw=1  action=0  varsize=off
  Multiport Switch2 : MultiPortSwitch  Inputs=2  zeroidx=on
  Relational Operator : RelationalOperator  Operator===  LogicOutDataTypeMode=boolean  OutDataTypeStr=boolean
  Terminator : Terminator
  att limits : Subsystem
  combine limits : Subsystem
  compute dc_fltpath : Subsystem
  throttle limits : Subsystem
  params : Outport  OutDataType=sfix(16)  OutScaling=2^0
  wires:
  Constant4/1 -> Bus Creator1/6  "wght_u_pref"
  Constant3/1 -> Bus Creator1/5  "u_pref"
  Multiport Switch2/1 -> Bus Creator1/7  "wght_cv"
  Constant1/1 -> Multiport Switch2/2
  full_surf/1 -> throttle limits/1(full_surf)
  Bus Selector/1 -> Bus Creator1/1  "<u_ulim>"
  Bus Selector/2 -> Bus Creator1/2  "<u_llim>"
  Bus Selector/4 -> Bus Creator1/4  "<u_lrlim>"
  Bus Creator1/1 -> params/1
  Relational Operator/1 -> Logical Operator/1
  Logical Operator/1 -> Multiport Switch2/1
  uvw/1 -> att limits/1(uvw)
  att limits/1(att_limits) -> combine limits/1(att_limits)
  throttle limits/1(throt_limits) -> combine limits/2(throt_limits), Bus Selector1/1
  combine limits/1(vel_u_limits) -> Bus Selector/1
  Bus Selector/3 -> Bus Creator1/3  "<u_urlim>"
  Bus Selector1/1 -> Relational Operator/1  "<throt_ulim>"
  Bus Selector1/2 -> Relational Operator/2  "<throt_llim>"
  Demux1/2 -> throttle limits/2(throt_old)
  Demux1/1 -> Terminator/1
  u_old/1 -> Demux1/1
  Gain2/1 -> Multiport Switch2/3
  NEh_dot_cmd/1 -> compute dc_fltpath/1(NEh_dot_fltpath)
  Manual Switch/1 -> Gain2/1
  dc_fltpath/1 -> Manual Switch/1
  compute dc_fltpath/1(dc_fltpath) -> Manual Switch/2

== system main_sim_adapt_Gref_SPPH/claw_main/vel_loops/to full att/e cmd ==
  d_cmd : Inport  OutDataType=sfix(16)  OutScaling=2^0
  cam : Inport  Port=2  OutDataType=sfix(16)  OutScaling=2^0
  Demux : Demux  Outputs=[ 2 MACH.num_u_throt ]
  Mux : Mux  Inputs=2
  Mux1 : Mux  Inputs=2
  Mux4 : Mux  Inputs=2
  att2e : utility_lib/att2e  SystemSampleTime=-1  quat_IC=MACH_quat_IC
  att,T : Outport  OutDataType=sfix(16)  OutScaling=2^0
  e,T : Outport  Port=2  OutDataType=sfix(16)  OutScaling=2^0
  wires:
  Demux/2 -> Mux/2, Mux1/2  "throt"
  Demux/1 -> Mux4/1
  cam/1 -> Mux4/2
  Mux4/1 -> Mux/1, att2e/1  "att"
  d_cmd/1 -> Demux/1
  Mux/1 -> att,T/1
  att2e/1 -> Mux1/1
  Mux1/1 -> e,T/1

== system main_sim_adapt_Gref_SPPH/claw_main/vel_loops/xu2d ==
  X : Inport  OutDataType=sfix(16)  OutScaling=2^0
  U : Inport  Port=2  OutDataType=sfix(16)  OutScaling=2^0
  params : Inport  Port=3  OutDataType=sfix(16)  OutScaling=2^0
  Assignment : Assignment  IndexOptions=Index vector (dialog)  Indices=MACH.throttle_idx  OutputSizes=[1 1]
  Bus Selector : BusSelector  OutputSignals=u_llim,u_ulim
  Demux : Demux  Outputs=[ 2 1 ]
  MinMax : MinMax  Inputs=2  OutDataType=sfix(16)  OutScaling=2^0  SaturateOnIntegerOverflow=on  InputSameDT=on
  MinMax1 : MinMax  Function=max  Inputs=2  OutDataType=sfix(16)  OutScaling=2^0  SaturateOnIntegerOverflow=on  InputSameDT=on
  Mux : Mux  Inputs=2
  Reshape : Reshape
  Selector1 : Selector  InputPortWidth=MACH.num_x  IndexOptions=Index vector (dialog)  Indices=MACH.quat_idx  OutputSizes=1
  Selector2 : Selector  InputPortWidth=MACH.num_u  IndexOptions=Index vector (dialog)  Indices=MACH.throttle_idx  OutputSizes=1
  Selector3 : Selector  InputPortWidth=MACH.vel_num_u  IndexOptions=Index vector (dialog)  Indices=3:MACH.vel_num_u  OutputSizes=1
  Selector4 : Selector  InputPortWidth=MACH.vel_num_u  IndexOptions=Index vector (dialog)  Indices=3:MACH.vel_num_u  OutputSizes=1
  e2att : utility_lib/e2att  SystemSampleTime=-1
  U_limited : Outport  OutDataType=sfix(16)  OutScaling=2^0
  d_nom : Outport  Port=2  OutDataType=sfix(16)  OutScaling=2^0
  cam : Outport  Port=3  OutDataType=sfix(16)  OutScaling=2^0
  wires:
  Selector1/1 -> e2att/1
  Selector2/1 -> MinMax1/1  "throttle"
  Mux/1 -> d_nom/1
  X/1 -> Selector1/1
  U/1 -> Selector2/1, Assignment/1
  Demux/1 -> Mux/1
  Demux/2 -> cam/1
  params/1 -> Bus Selector/1
  Bus Selector/1 -> Selector3/1  "<u_llim>"
  MinMax1/1 -> MinMax/1
  Bus Selector/2 -> Selector4/1  "<u_ulim>"
  Selector4/1 -> MinMax/2
  Selector3/1 -> MinMax1/2
  MinMax/1 -> Assignment/2, Reshape/1
  Assignment/1 -> U_limited/1
  e2att/1 -> Demux/1
  Reshape/1 -> Mux/2

== system main_sim_adapt_Gref_SPPH/control input (modified)/Add Excitation/Excitation  Signal ==
  Enable : EnablePort  StatesWhenEnabling=reset  ShowOutputPort=on
  Lookup Table1 : Lookup  InputValues=in_exsig_vecin  Table=in_exsig_vecout  LookUpMeth=Use Input Above  OutDataType=sfix(16)  OutScaling=2^0
  excitaiton output sig : Scope
      settings: TimeRange=45  YMin=-0.05  YMax=0.05  SaveName=ScopeData5
  excitation input sig : Scope
      settings: TimeRange=45  YMin=15  YMax=22  SaveName=ScopeData10
  int_Kxhat1 : DiscreteIntegrator  ExternalReset=falling  SampleTime=-1  OutDataType=sfix(16)  OutScaling=2^0  ICPrevOutput=DiscIntNeverNeededParam  ICPrevScaledInput=DiscIntNeverNeededParam
  exsig : Outport  OutDataType=sfix(16)  OutScaling=2^0  OutputWhenDisabled=reset  InitialOutput=0
  wires:
  Lookup Table1/1 -> exsig/1, excitaiton output sig/1
  Enable/1 -> int_Kxhat1/2, int_Kxhat1/1
  int_Kxhat1/1 -> Lookup Table1/1, excitation input sig/1

== system main_sim_adapt_Gref_SPPH/control input (modified)/control input/form control input ==
  cmd_bus : Inport  OutDataType=sfix(16)  OutScaling=2^0
  Bus Creator : BusCreator
  Bus Selector4 : BusSelector  OutputSignals=command,full_surf_cmd
  add effector control params : Subsystem
  engine parameters : Subsystem
  mode switches : Subsystem
  select command : Subsystem
  control_input : Outport  OutDataType=sfix(16)  OutScaling=2^0
  wires:
  select command/1(control_input) -> Bus Selector4/1, mode switches/1(control_input)
  Bus Selector4/1 -> Bus Creator/1  "<command>"
  add effector control params/1(full_surf) -> Bus Creator/2  "full_surf"
  Bus Selector4/2 -> add effector control params/1(full_surf_cmd)  "<full_surf_cmd>"
  engine parameters/1(engines) -> Bus Creator/4  "engines"
  mode switches/1(mode_sw) -> Bus Creator/3  "mode_sw"
  cmd_bus/1 -> select command/1(cmd_bus)
  Bus Creator/1 -> control_input/1

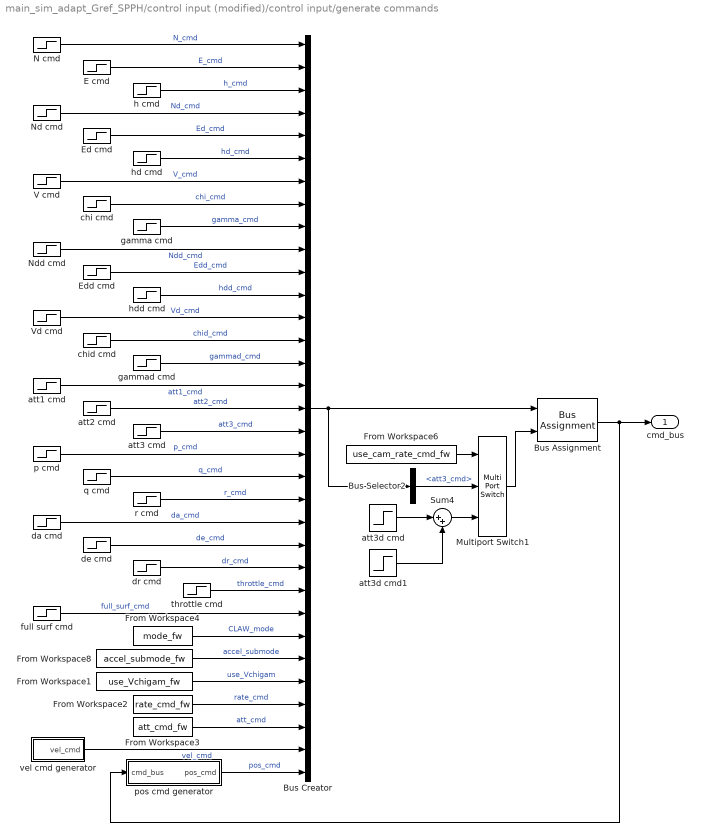
== system main_sim_adapt_Gref_SPPH/control input (modified)/control input/generate commands ==
  Bus Assignment : BusAssignment  AssignedSignals=att3_cmd
  Bus Creator : BusCreator  Inputs=33
  Bus Selector2 : BusSelector  OutputSignals=att3_cmd
  E cmd : Step  Time=command_time  Before=E_trim_IC  After=E_trim_IC+10*0  SampleTime=MACH.dt
  Ed cmd : Step  Time=command_time  Before=Ed_trim_IC  After=Ed_trim_IC  SampleTime=MACH.dt
  Edd cmd : Step  Time=command_time  After=0  SampleTime=MACH.dt
  From Workspace1 : FromWorkspace  VariableName=use_Vchigam_fw  SampleTime=MACH.dt  Interpolate=off  OutputAfterFinalValue=Holding final value
  From Workspace2 : FromWorkspace  VariableName=rate_cmd_fw  SampleTime=MACH.dt  OutputAfterFinalValue=Holding final value
  From Workspace3 : FromWorkspace  VariableName=att_cmd_fw  SampleTime=MACH.dt  OutputAfterFinalValue=Holding final value
  From Workspace4 : FromWorkspace  VariableName=mode_fw  SampleTime=MACH.dt  Interpolate=off  OutputAfterFinalValue=Holding final value
  From Workspace6 : FromWorkspace  VariableName=use_cam_rate_cmd_fw  SampleTime=MACH.dt  Interpolate=off  OutputAfterFinalValue=Holding final value
  From Workspace8 : FromWorkspace  VariableName=accel_submode_fw  SampleTime=MACH.dt  Interpolate=off  OutputAfterFinalValue=Holding final value
  Multiport Switch1 : MultiPortSwitch  Inputs=2  zeroidx=on
  N cmd : Step  Time=command_time  Before=N_trim_IC  After=N_trim_IC+10*0  SampleTime=MACH.dt
  Nd cmd : Step  Time=command_time  Before=Nd_trim_IC  After=Nd_trim_IC  SampleTime=MACH.dt
  Ndd cmd : Step  Time=command_time  After=0  SampleTime=MACH.dt
  Sum4 : Sum  Inputs=|++  OutDataType=sfix(16)  OutScaling=2^0  SaturateOnIntegerOverflow=on
  V cmd : Step  Time=command_time  Before=V_trim_IC  After=V_trim_IC  SampleTime=MACH.dt
  Vd cmd : Step  Time=command_time  After=0  SampleTime=MACH.dt
  att1 cmd : Step  Tag=tilta  Time=command_time  Before=att_trim_IC(1)  After=att_trim_IC(1) + 0.1*0  SampleTime=MACH.dt
      settings: AttributesFormatString=%<Name> (%<Tag>)
  att2 cmd : Step  Tag=tiltb  Description=theta  Time=command_time  Before=att_trim_IC(2)  After="att_trim_IC(2)  + 0.1*0"  SampleTime=MACH.dt
      settings: AttributesFormatString=%<Name> (%<Tag>)
  att3 cmd : Step  Tag=cam  Time=command_time  Before=att_trim_IC(3)  After="att_trim_IC(3)  + 0.1*0"  SampleTime=MACH.dt
      settings: AttributesFormatString=%<Name> (%<Tag>)
  att3d cmd : Step  Tag=cam  Time=command_time + (15 - command_time)  After=-0.04*0  SampleTime=MACH.dt
      settings: AttributesFormatString=%<Name> (%<Tag>)
  att3d cmd1 : Step  Time=command_time + (17 - command_time)  After=0.04*0  SampleTime=MACH.dt
  chi cmd : Step  Time=command_time  Before=chi_trim_IC  After=chi_trim_IC  SampleTime=MACH.dt
  chid cmd : Step  Time=command_time  After=0  SampleTime=MACH.dt
  da cmd : Step  Time=command_time  Before=da_trim_IC  After=da_trim_IC  SampleTime=MACH.dt
  de cmd : Step  Time=command_time  Before=de_trim_IC  After=de_trim_IC  SampleTime=MACH.dt
  dr cmd : Step  Time=command_time  Before=dr_trim_IC  After=dr_trim_IC  SampleTime=MACH.dt
  full surf cmd : Step  Time=command_time  Before=MACH_U_nom_IC  After=MACH_U_nom_IC  SampleTime=MACH.dt
  gamma cmd : Step  Time=command_time  Before=gamma_trim_IC  After=gamma_trim_IC  SampleTime=MACH.dt
  gammad cmd : Step  Time=command_time  After=0  SampleTime=MACH.dt
  h cmd : Step  Time=command_time  Before=h_trim_IC  After=h_trim_IC + 10*0  SampleTime=MACH.dt
  hd cmd : Step  Time=command_time  Before=hd_trim_IC  After=hd_trim_IC  SampleTime=MACH.dt
  hdd cmd : Step  Time=command_time  After=0  SampleTime=MACH.dt
  p cmd : Step  Time=command_time  Before=pqr_trim_IC(1)  After=pqr_trim_IC(1) + 0.2*0  SampleTime=MACH.dt
  pos cmd generator : Subsystem
  q cmd : Step  Time=command_time  Before=pqr_trim_IC(2)  After=pqr_trim_IC(2) + 0.2*0  SampleTime=MACH.dt
  r cmd : Step  Time=command_time  Before=pqr_trim_IC(3)  After=pqr_trim_IC(3) + 0.2*0  SampleTime=MACH.dt
  throttle cmd : Step  Time=command_time  Before=throttle_trim_IC(1)  After=throttle_trim_IC(1)  SampleTime=MACH.dt
  vel cmd generator : Subsystem
  cmd_bus : Outport  OutDataType=sfix(16)  OutScaling=2^0
  wires:
  From Workspace2/1 -> Bus Creator/30  "rate_cmd"
  From Workspace1/1 -> Bus Creator/29  "use_Vchigam"
  gamma cmd/1 -> Bus Creator/9  "gamma_cmd"
  chi cmd/1 -> Bus Creator/8  "chi_cmd"
  V cmd/1 -> Bus Creator/7  "V_cmd"
  gammad cmd/1 -> Bus Creator/15  "gammad_cmd"
  chid cmd/1 -> Bus Creator/14  "chid_cmd"
  Vd cmd/1 -> Bus Creator/13  "Vd_cmd"
  hdd cmd/1 -> Bus Creator/12  "hdd_cmd"
  Edd cmd/1 -> Bus Creator/11  "Edd_cmd"
  Ndd cmd/1 -> Bus Creator/10  "Ndd_cmd"
  full surf cmd/1 -> Bus Creator/26  "full_surf_cmd"
  From Workspace8/1 -> Bus Creator/28  "accel_submode"
  From Workspace4/1 -> Bus Creator/27  "CLAW_mode"
  pos cmd generator/1(pos_cmd) -> Bus Creator/33  "pos_cmd"
  vel cmd generator/1(vel_cmd) -> Bus Creator/32  "vel_cmd"
  From Workspace3/1 -> Bus Creator/31  "att_cmd"
  Bus Assignment/1 -> cmd_bus/1, pos cmd generator/1(cmd_bus)
  Multiport Switch1/1 -> Bus Assignment/2
  Bus Selector2/1 -> Multiport Switch1/2  "<att3_cmd>"
  att3d cmd1/1 -> Sum4/2
  att3d cmd/1 -> Sum4/1
  Sum4/1 -> Multiport Switch1/3
  From Workspace6/1 -> Multiport Switch1/1
  N cmd/1 -> Bus Creator/1  "N_cmd"
  E cmd/1 -> Bus Creator/2  "E_cmd"
  h cmd/1 -> Bus Creator/3  "h_cmd"
  Nd cmd/1 -> Bus Creator/4  "Nd_cmd"
  Ed cmd/1 -> Bus Creator/5  "Ed_cmd"
  hd cmd/1 -> Bus Creator/6  "hd_cmd"
  att1 cmd/1 -> Bus Creator/16  "att1_cmd"
  att2 cmd/1 -> Bus Creator/17  "att2_cmd"
  att3 cmd/1 -> Bus Creator/18  "att3_cmd"
  p cmd/1 -> Bus Creator/19  "p_cmd"
  q cmd/1 -> Bus Creator/20  "q_cmd"
  r cmd/1 -> Bus Creator/21  "r_cmd"
  da cmd/1 -> Bus Creator/22  "da_cmd"
  de cmd/1 -> Bus Creator/23  "de_cmd"
  dr cmd/1 -> Bus Creator/24  "dr_cmd"
  throttle cmd/1 -> Bus Creator/25  "throttle_cmd"
  Bus Creator/1 -> Bus Selector2/1, Bus Assignment/1
